simulink model "second"  (R2024a)
settings: Solver=VariableStepAuto  StartTime=0.0  StopTime=5  RelTol=1e-3
values from neighbouring files (symbols this model uses):
  A = 5    [third_calc.m]
  B = 5.5    [third_calc.m]
  T = 0.2    [first_calc.m]    (also in second.m; third_calc.m = 0.25)
undefined symbols (not defined in the file or in its folder): K1, K2, K3, K4, K5, x0
settings Model: Creator=ventus  LastModifiedBy=ventus

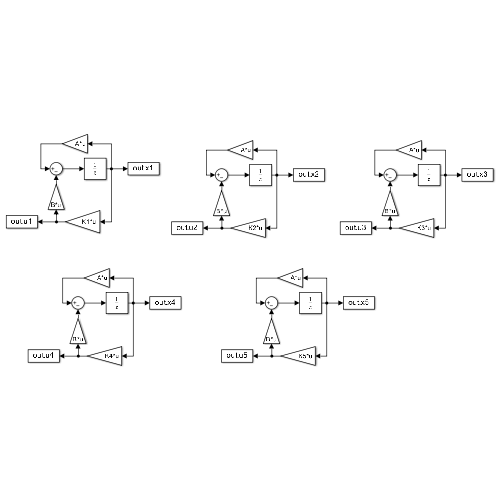
[thumbnail: Simulink's stored preview of the top-level diagram]
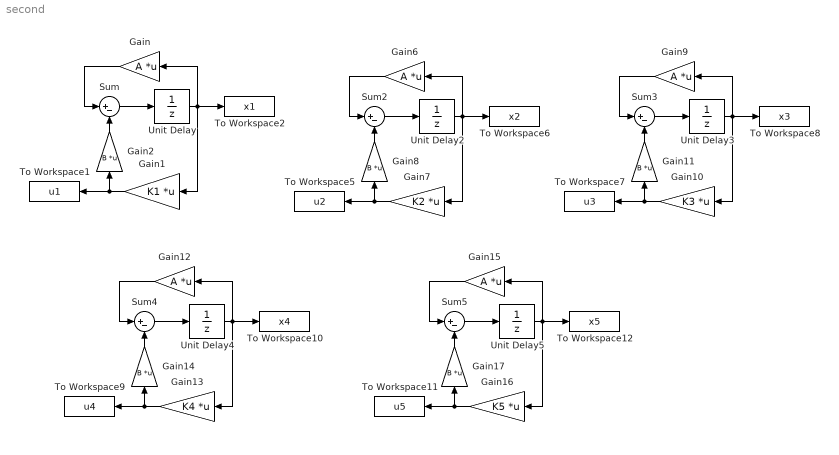
== system second ==
  Gain{,6,9,12,15} (5 alike) : Gain  Gain=A  Multiplication=Matrix(K*u)
  Gain1 : Gain  Gain=K1  Multiplication=Matrix(K*u)
  Gain10 : Gain  Gain=K3  Multiplication=Matrix(K*u)
  Gain{2,8,11,14,17} (5 alike) : Gain  Gain=B  Multiplication=Matrix(K*u)
  Gain13 : Gain  Gain=K4  Multiplication=Matrix(K*u)
  Gain16 : Gain  Gain=K5  Multiplication=Matrix(K*u)
  Gain7 : Gain  Gain=K2  Multiplication=Matrix(K*u)
  Sum{,2..5} (5 alike) : Sum  Inputs=|+-
  To Workspace1 : ToWorkspace  VariableName=u1  SaveFormat=Timeseries  SampleTime=-1
  To Workspace10 : ToWorkspace  VariableName=x4  SaveFormat=Timeseries  SampleTime=-1
  To Workspace11 : ToWorkspace  VariableName=u5  SaveFormat=Timeseries  SampleTime=-1
  To Workspace12 : ToWorkspace  VariableName=x5  SaveFormat=Timeseries  SampleTime=-1
  To Workspace2 : ToWorkspace  VariableName=x1  SaveFormat=Timeseries  SampleTime=-1
  To Workspace5 : ToWorkspace  VariableName=u2  SaveFormat=Timeseries  SampleTime=-1
  To Workspace6 : ToWorkspace  VariableName=x2  SaveFormat=Timeseries  SampleTime=-1
  To Workspace7 : ToWorkspace  VariableName=u3  SaveFormat=Timeseries  SampleTime=-1
  To Workspace8 : ToWorkspace  VariableName=x3  SaveFormat=Timeseries  SampleTime=-1
  To Workspace9 : ToWorkspace  VariableName=u4  SaveFormat=Timeseries  SampleTime=-1
  Unit Delay{,2..5} (5 alike) : UnitDelay  InitialCondition=x0  SampleTime=T  HasFrameUpgradeWarning=on
  wires:
  Sum/1 -> Unit Delay/1
  Gain/1 -> Sum/1
  Unit Delay/1 -> To Workspace2/1, Gain1/1, Gain/1
  Gain1/1 -> Gain2/1, To Workspace1/1
  Gain2/1 -> Sum/2
  Gain7/1 -> Gain8/1, To Workspace5/1
  Gain8/1 -> Sum2/2
  Unit Delay2/1 -> To Workspace6/1, Gain7/1, Gain6/1
  Sum2/1 -> Unit Delay2/1
  Gain6/1 -> Sum2/1
  Gain10/1 -> Gain11/1, To Workspace7/1
  Gain11/1 -> Sum3/2
  Unit Delay3/1 -> To Workspace8/1, Gain10/1, Gain9/1
  Sum3/1 -> Unit Delay3/1
  Gain9/1 -> Sum3/1
  Gain13/1 -> Gain14/1, To Workspace9/1
  Gain14/1 -> Sum4/2
  Unit Delay4/1 -> To Workspace10/1, Gain13/1, Gain12/1
  Sum4/1 -> Unit Delay4/1
  Gain12/1 -> Sum4/1
  Gain16/1 -> Gain17/1, To Workspace11/1
  Gain17/1 -> Sum5/2
  Unit Delay5/1 -> To Workspace12/1, Gain16/1, Gain15/1
  Sum5/1 -> Unit Delay5/1
  Gain15/1 -> Sum5/1
